simulink model "topavalon"  (Simulink 7.0)
settings: Solver=FixedStepDiscrete  StartTime=0.0  StopTime=100.0  FixedStep=1  RelTol=1e-3
InitFcn:
  | %% DSPBuilder Start
  | alt_dspbuilder_update_model(bdroot)
  | %% DSPBuilder End
undefined symbols (not defined in the file): Pin_U10, Pin_U11, Pin_U5, Pin_U6, Pin_V10, Pin_V4, Pin_V5, Pin_V6, Pin_V7, Pin_V9, Pin_W6, Pin_W7, Pin_W8, Pin_W9
libraries: allblocks_alteradspbuilder2 x33, Stratix_EP2S60_alteradspbuilder2 x3, simulink x2
settings Model: Creator=DOLSEN  LastModifiedBy=DOLSEN
settings DataIOCC: SignalLoggingName=sigsOut
settings OptimizationCC: BlockReduction=off  BooleanDataType=off
settings DebuggingCC: AlgebraicLoopMsg=none  SaveWithParameterizedLinksMsg=none  SignalResolutionControl=TryResolveAllWithWarning  SolverPrmCheckMsg=none  MultiTaskDSMMsg=warning  MultiTaskCondExecSysMsg=none
settings HardwareCC: TargetUnknown=on
settings RTWCC: IncludeERTFirstTime=on
settings GRTTargetCC: TargetFcnLib=ansi_tfl_tmw.mat  ModelReferenceCompliant=off  MatFileLogging=off

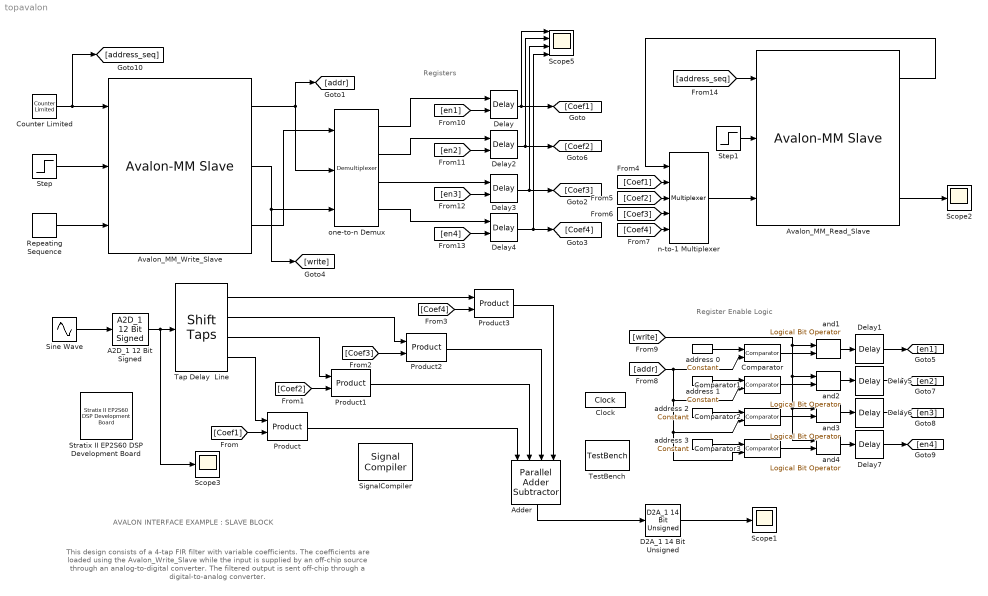
== system topavalon ==
  note: AVALON INTERFACE EXAMPLE : SLAVE BLOCK
  note: This design consists of a 4-tap FIR filter with variable coefficients.  The
      | coefficients are loaded using the Avalon_Write_Slave while the input is
      | supplied by an off-chip source through an analog-to-digital converter. The
      | filtered output is sent off-chip through a digital-to-analog converter.
  note: Register Enable Logic
  note: Registers
  A2D_1 12 Bit Signed : Stratix_EP2S60_alteradspbuilder2/A2D_1 12 Bit Signed  iofile=C:\altera\80\quartus\dsp_builder\DesignExamples\Tutorials\SOPCBuilder\SOPCBlock\My_System\tb_topavalon\topavalon_A2D%5F1+12+Bit+Signed.salt  externalType=Inferred  SpecifyClock=off  location=Pin_D1,Pin_D2 ,Pin_E3 ,Pin_E4 ,Pin_E1 ,Pin_E2 ,Pin_F3 ,Pin_F4 ,Pin_F1 ,Pin_F2 ,Pin_G3 ,Pin_G4
  Adder : allblocks_alteradspbuilder2/Parallel Adder Subtractor  Orientation=down  number_of_inputs=4  direction=++  use_pipeline=off  pipeline_display=0  phase_selection=1  use_ena=off  use_aclr=off  allowFloatingPointOverride=on  logOutputs=off  logFile=C:\altera\80\quartus\dsp_builder\DesignExamples\Tutorials\SOPCBuilder\SOPCBlock\My_System\tb_topavalon\topavalon_Adder.fixedpointlog
  Avalon_MM_Read_Slave : allblocks_alteradspbuilder2/Avalon-MM Slave  SystemSampleTime=-1  iofile=C:\altera\80\quartus\dsp_builder\DesignExamples\Tutorials\SOPCBuilder\SOPCBlock\My_System\tb_topavalon\topavalon_Avalon%5FMM%5FRead%5FSlave_address.salt,C:\altera\80\quartus\dsp_builder\DesignExamples\Tutorials\SOPCBuilder\SOPCBlock\My_System\tb_topavalon\topavalon_Avalon%5FMM%5FRead%5FSlave_read.salt,C:\altera\80\quartus\dsp_builder\DesignExamples\Tutorials\SOPCBuilder\SOPCBlock\My_System\tb_topavalon\topavalon_Avalon%5FMM%5FRead%5FSlave_readdata.capture,  SpecifyClock=off  addrWidth=2  addrAlignment=Dynamic  addrType=Read  BusType=Unsigned Integer  bwl=8  bwr=0  byteEnable=off  flowCtrl=off  pipeline=off  waitStateFormat=Fixed  readWaitStateCycles=0  writeWaitStateCycles=0  readLatencyFormat=Fixed  readLatencyCycles=0  burst=off  maxBurst=4  irq=off  receiveBeginTransfer=off  useChipSelect=off  externalType=Inferred  PORTTYPE=Output
  Avalon_MM_Write_Slave : allblocks_alteradspbuilder2/Avalon-MM Slave  SystemSampleTime=-1  iofile=C:\altera\80\quartus\dsp_builder\DesignExamples\Tutorials\SOPCBuilder\SOPCBlock\My_System\tb_topavalon\topavalon_Avalon%5FMM%5FWrite%5FSlave_address.salt,C:\altera\80\quartus\dsp_builder\DesignExamples\Tutorials\SOPCBuilder\SOPCBlock\My_System\tb_topavalon\topavalon_Avalon%5FMM%5FWrite%5FSlave_write.salt,C:\altera\80\quartus\dsp_builder\DesignExamples\Tutorials\SOPCBuilder\SOPCBlock\My_System\tb_topavalon\topavalon_Avalon%5FMM%5FWrite%5FSlave_writedata.salt,  SpecifyClock=off  addrWidth=2  addrAlignment=Dynamic  addrType=Write  BusType=Unsigned Integer  bwl=8  bwr=0  byteEnable=off  flowCtrl=off  pipeline=off  waitStateFormat=Fixed  readWaitStateCycles=0  writeWaitStateCycles=0  readLatencyFormat=Fixed  readLatencyCycles=0  burst=off  maxBurst=4  irq=off  receiveBeginTransfer=off  useChipSelect=off  externalType=Inferred  PORTTYPE=Output
  Clock : allblocks_alteradspbuilder2/Clock  ClockPeriod=100  ClockPeriodUnit=ns  SampleTime=1  SimulationStartCycle=5  PhaseOffset=0  Reset=aclr  ResetType=Active Low  Export=off
  Comparator : allblocks_alteradspbuilder2/Comparator  direction=a == b  pipeline_display=0  allowFloatingPointOverride=on  logOutputs=off  logFile=C:\altera\80\quartus\dsp_builder\DesignExamples\Tutorials\SOPCBuilder\SOPCBlock\My_System\tb_topavalon\topavalon_Comparator.fixedpointlog
  Comparator1 : allblocks_alteradspbuilder2/Comparator  direction=a == b  pipeline_display=0  allowFloatingPointOverride=on  logOutputs=off  logFile=C:\altera\80\quartus\dsp_builder\DesignExamples\Tutorials\SOPCBuilder\SOPCBlock\My_System\tb_topavalon\topavalon_Comparator1.fixedpointlog
  Comparator2 : allblocks_alteradspbuilder2/Comparator  direction=a == b  pipeline_display=0  allowFloatingPointOverride=on  logOutputs=off  logFile=C:\altera\80\quartus\dsp_builder\DesignExamples\Tutorials\SOPCBuilder\SOPCBlock\My_System\tb_topavalon\topavalon_Comparator2.fixedpointlog
  Comparator3 : allblocks_alteradspbuilder2/Comparator  direction=a == b  pipeline_display=0  allowFloatingPointOverride=on  logOutputs=off  logFile=C:\altera\80\quartus\dsp_builder\DesignExamples\Tutorials\SOPCBuilder\SOPCBlock\My_System\tb_topavalon\topavalon_Comparator3.fixedpointlog
  Counter Limited : simulink/Sources/Counter Limited  SystemSampleTime=-1  uplimit=3  tsamp=1
  D2A_1 14 Bit Unsigned : Stratix_EP2S60_alteradspbuilder2/D2A_1 14 Bit Unsigned  iofile=C:\altera\80\quartus\dsp_builder\DesignExamples\Tutorials\SOPCBuilder\SOPCBlock\My_System\tb_topavalon\topavalon_D2A%5F1+14+Bit+Unsigned.capture  externalType=Inferred  location=Pin_W7,Pin_W6,Pin_W9,Pin_W8,Pin_V5,Pin_V4,Pin_V7,Pin_V6,Pin_V10,Pin_V9,Pin_U11,Pin_U10,Pin_U6,Pin_U5
  Delay : allblocks_alteradspbuilder2/Delay  pipeline=1  pipeline_display=1  ClockPhase=1  use_ena=on  use_sclr=off  allowFloatingPointOverride=on  logOutputs=off  logFile=C:\altera\80\quartus\dsp_builder\DesignExamples\Tutorials\SOPCBuilder\SOPCBlock\My_System\tb_topavalon\topavalon_Delay.fixedpointlog  use_init=off  reset_value=1
  Delay1 : allblocks_alteradspbuilder2/Delay  pipeline=1  pipeline_display=1  ClockPhase=1  use_ena=off  use_sclr=off  allowFloatingPointOverride=on  logOutputs=off  logFile=C:\altera\80\quartus\dsp_builder\DesignExamples\Tutorials\SOPCBuilder\SOPCBlock\My_System\tb_topavalon\topavalon_Delay1.fixedpointlog  use_init=off  reset_value=1
  Delay2 : allblocks_alteradspbuilder2/Delay  pipeline=1  pipeline_display=1  ClockPhase=1  use_ena=on  use_sclr=off  allowFloatingPointOverride=on  logOutputs=off  logFile=C:\altera\80\quartus\dsp_builder\DesignExamples\Tutorials\SOPCBuilder\SOPCBlock\My_System\tb_topavalon\topavalon_Delay2.fixedpointlog  use_init=off  reset_value=1
  Delay3 : allblocks_alteradspbuilder2/Delay  pipeline=1  pipeline_display=1  ClockPhase=1  use_ena=on  use_sclr=off  allowFloatingPointOverride=on  logOutputs=off  logFile=C:\altera\80\quartus\dsp_builder\DesignExamples\Tutorials\SOPCBuilder\SOPCBlock\My_System\tb_topavalon\topavalon_Delay3.fixedpointlog  use_init=off  reset_value=1
  Delay4 : allblocks_alteradspbuilder2/Delay  pipeline=1  pipeline_display=1  ClockPhase=1  use_ena=on  use_sclr=off  allowFloatingPointOverride=on  logOutputs=off  logFile=C:\altera\80\quartus\dsp_builder\DesignExamples\Tutorials\SOPCBuilder\SOPCBlock\My_System\tb_topavalon\topavalon_Delay4.fixedpointlog  use_init=off  reset_value=1
  Delay5 : allblocks_alteradspbuilder2/Delay  pipeline=1  pipeline_display=1  ClockPhase=1  use_ena=off  use_sclr=off  allowFloatingPointOverride=on  logOutputs=off  logFile=C:\altera\80\quartus\dsp_builder\DesignExamples\Tutorials\SOPCBuilder\SOPCBlock\My_System\tb_topavalon\topavalon_Delay5.fixedpointlog  use_init=off  reset_value=1
  Delay6 : allblocks_alteradspbuilder2/Delay  pipeline=1  pipeline_display=1  ClockPhase=1  use_ena=off  use_sclr=off  allowFloatingPointOverride=on  logOutputs=off  logFile=C:\altera\80\quartus\dsp_builder\DesignExamples\Tutorials\SOPCBuilder\SOPCBlock\My_System\tb_topavalon\topavalon_Delay6.fixedpointlog  use_init=off  reset_value=1
  Delay7 : allblocks_alteradspbuilder2/Delay  pipeline=1  pipeline_display=1  ClockPhase=1  use_ena=off  use_sclr=off  allowFloatingPointOverride=on  logOutputs=off  logFile=C:\altera\80\quartus\dsp_builder\DesignExamples\Tutorials\SOPCBuilder\SOPCBlock\My_System\tb_topavalon\topavalon_Delay7.fixedpointlog  use_init=off  reset_value=1
  Product : allblocks_alteradspbuilder2/Product  BusType=Inferred  bwl=8  bwr=0  pipeline=0  pipeline_display=0  phase_selection=1  use_ena=off  use_aclr=off  UseLPM=off  UseDedicatedCircuitry=off  allowFloatingPointOverride=on  logOutputs=off  logFile=C:\altera\80\quartus\dsp_builder\DesignExamples\Tutorials\SOPCBuilder\SOPCBlock\My_System\tb_topavalon\topavalon_Product.fixedpointlog
  Product1 : allblocks_alteradspbuilder2/Product  BusType=Inferred  bwl=8  bwr=0  pipeline=0  pipeline_display=0  phase_selection=1  use_ena=off  use_aclr=off  UseLPM=off  UseDedicatedCircuitry=off  allowFloatingPointOverride=on  logOutputs=off  logFile=C:\altera\80\quartus\dsp_builder\DesignExamples\Tutorials\SOPCBuilder\SOPCBlock\My_System\tb_topavalon\topavalon_Product1.fixedpointlog
  Product2 : allblocks_alteradspbuilder2/Product  BusType=Inferred  bwl=8  bwr=0  pipeline=0  pipeline_display=0  phase_selection=1  use_ena=off  use_aclr=off  UseLPM=off  UseDedicatedCircuitry=off  allowFloatingPointOverride=on  logOutputs=off  logFile=C:\altera\80\quartus\dsp_builder\DesignExamples\Tutorials\SOPCBuilder\SOPCBlock\My_System\tb_topavalon\topavalon_Product2.fixedpointlog
  Product3 : allblocks_alteradspbuilder2/Product  BusType=Inferred  bwl=8  bwr=0  pipeline=0  pipeline_display=0  phase_selection=1  use_ena=off  use_aclr=off  UseLPM=off  UseDedicatedCircuitry=off  allowFloatingPointOverride=on  logOutputs=off  logFile=C:\altera\80\quartus\dsp_builder\DesignExamples\Tutorials\SOPCBuilder\SOPCBlock\My_System\tb_topavalon\topavalon_Product3.fixedpointlog
  Repeating Sequence : simulink/Sources/Repeating Sequence  SystemSampleTime=-1  rep_seq_t=[0 1 2 3 4]  rep_seq_y=[1 0 0 0 0]
  Scope1 : Scope
      settings: SampleInput=on
  Scope2 : Scope
      settings: SampleInput=on
  Scope3 : Scope
      settings: SaveName=ScopeData2  SampleInput=on
  Scope5 : Scope  NumInputPorts=4
      settings: TimeRange=100  YMin=0~0~0~-1  YMax=1~1~1~1  SaveName=ScopeData3  SampleInput=on
  SignalCompiler : allblocks_alteradspbuilder2/Signal Compiler  DeviceFamily=Stratix II  DeviceName=EP2S60F1020C4ES  EnableSignalTap=off  SignalTapDepth=128  UseBoardBlock=off  StpUseDefaultClock=on  StpClock=Clock  ExportDir=C:\Documents and Settings\dolsen\My Documents
  Sine Wave : Sin  Amplitude=2^11-1  SampleTime=1
  Step : Step  Time=4  Before=1  After=0  SampleTime=1
  Step1 : Step  Time=10  Before=1  After=0  SampleTime=1
  Stratix II EP2S60 DSP Development Board : Stratix_EP2S60_alteradspbuilder2/Stratix II EP2S60 DSP Development Board  ClockPinIn=Pin_AM17  GlobalResetPin=Pin_AG19  device=EP2S60F1020C4
  Tap Delay  Line : allblocks_alteradspbuilder2/Shift Taps  number_of_taps=4  tap_distance=1  use_shiftout=off  use_ena=off  use_sclr=off  use_dedicated_circuitry=on  ram_type=AUTO  allowFloatingPointOverride=on  logOutputs=off  logFile=C:\altera\80\quartus\dsp_builder\DesignExamples\Tutorials\SOPCBuilder\SOPCBlock\My_System\tb_topavalon\topavalon_Tap+Delay+%0ALine%3A%3At.fixedpointlog,C:\altera\80\quartus\dsp_builder\DesignExamples\Tutorials\SOPCBuilder\SOPCBlock\My_System\tb_topavalon\topavalon_Tap+Delay+%0ALine%3A%3At.fixedpointlog,C:\altera\80\quartus\dsp_builder\DesignExamples\Tutorials\SOPCBuilder\SOPCBlock\My_System\tb_topavalon\topavalon_Tap+Delay+%0ALine%3A%3At.fixedpointlog,C:\altera\80\quartus\dsp_builder\DesignExamples\Tutorials\SOPCBuilder\SOPCBlock\My_System\tb_topavalon\topavalon_Tap+Delay+%0ALine%3A%3At.fixedpointlog,
  TestBench : allblocks_alteradspbuilder2/TestBench  enable=on  advancedMode=off  modelSimGui=off  maxDisplayErrors=10  mismatchErrorLevel=Error  simdatafile=C:\altera\80\quartus\dsp_builder\DesignExamples\Tutorials\SOPCBuilder\SOPCBlock\My_System\tb_topavalon\topavalon.simdata.tcl
  address 0 : allblocks_alteradspbuilder2/Constant  mask_cst=0  BusType=Unsigned Integer  bwl=2  bwr=0  roundMode=Truncate  satMode=Wrap  SpecifyClock=off  allowFloatingPointOverride=on  logOutputs=off  logFile=C:\altera\80\quartus\dsp_builder\DesignExamples\Tutorials\SOPCBuilder\SOPCBlock\My_System\tb_topavalon\topavalon_address+0.fixedpointlog
  address 1 : allblocks_alteradspbuilder2/Constant  mask_cst=1  BusType=Unsigned Integer  bwl=2  bwr=0  roundMode=Truncate  satMode=Wrap  SpecifyClock=off  allowFloatingPointOverride=on  logOutputs=off  logFile=C:\altera\80\quartus\dsp_builder\DesignExamples\Tutorials\SOPCBuilder\SOPCBlock\My_System\tb_topavalon\topavalon_address+1.fixedpointlog
  address 2 : allblocks_alteradspbuilder2/Constant  mask_cst=2  BusType=Unsigned Integer  bwl=2  bwr=0  roundMode=Truncate  satMode=Wrap  SpecifyClock=off  allowFloatingPointOverride=on  logOutputs=off  logFile=C:\altera\80\quartus\dsp_builder\DesignExamples\Tutorials\SOPCBuilder\SOPCBlock\My_System\tb_topavalon\topavalon_address+2.fixedpointlog
  address 3 : allblocks_alteradspbuilder2/Constant  mask_cst=3  BusType=Unsigned Integer  bwl=2  bwr=0  roundMode=Truncate  satMode=Wrap  SpecifyClock=off  allowFloatingPointOverride=on  logOutputs=off  logFile=C:\altera\80\quartus\dsp_builder\DesignExamples\Tutorials\SOPCBuilder\SOPCBlock\My_System\tb_topavalon\topavalon_address+3.fixedpointlog
  and{1..4} (4 alike) : allblocks_alteradspbuilder2/Logical Bit Operator  LogicalOperator=AND  user_inputs=2  pipeline_display=0
  n-to-1 Multiplexer : allblocks_alteradspbuilder2/Multiplexer  numInputs=4  pipeline=0  oneHot=off  pipeline_display=0  use_ena=off  use_aclr=off  allowFloatingPointOverride=on  logOutputs=off  logFile=C:\altera\80\quartus\dsp_builder\DesignExamples\Tutorials\SOPCBuilder\SOPCBlock\My_System\tb_topavalon\topavalon_n-to-1+Multiplexer.fixedpointlog
  one-to-n Demux : allblocks_alteradspbuilder2/Demultiplexer  numOutputs=4  pipeline_display=1  use_ena=on  use_sclr=off  allowFloatingPointOverride=on  logOutputs=off  logFile=C:\altera\80\quartus\dsp_builder\DesignExamples\Tutorials\SOPCBuilder\SOPCBlock\My_System_\tb_topavalon\topavalon_one-to-n+Demux%3A%3Aq.fixedpointlog,C:\altera\80\quartus\dsp_builder\DesignExamples\Tutorials\SOPCBuilder\SOPCBlock\My_System_\tb_topavalon\topavalon_one-to-n+Demux%3A%3Aq.fixedpointlog,C:\altera\80\quartus\dsp_builder\DesignExamples\Tutorials\SOPCBuilder\SOPCBlock\My_System_\tb_topavalon\topavalon_one-to-n+Demux%3A%3Aq.fixedpointlog,C:\altera\80\quartus\dsp_builder\DesignExamples\Tutorials\SOPCBuilder\SOPCBlock\My_System_\tb_topavalon\topavalon_one-to-n+Demux%3A%3Aq.fixedpointlog,
  wires:
  Tap Delay  Line/4 -> Product/1
  Tap Delay  Line/3 -> Product1/1
  Tap Delay  Line/2 -> Product2/1
  Tap Delay  Line/1 -> Product3/1
  Product/1 -> Adder/1
  A2D_1 12 Bit Signed/1 -> Tap Delay  Line/1, Scope3/1
  Product1/1 -> Adder/2
  Product2/1 -> Adder/3
  Product3/1 -> Adder/4
  Adder/1 -> D2A_1 14 Bit Unsigned/1
  [Coef1] -> Product/2
  [Coef2] -> Product1/2
  [Coef3] -> Product2/2
  [Coef4] -> Product3/2
  one-to-n Demux/1 -> Delay/1
  one-to-n Demux/2 -> Delay2/1
  one-to-n Demux/3 -> Delay3/1
  one-to-n Demux/4 -> Delay4/1
  Avalon_MM_Write_Slave/1 -> one-to-n Demux/2, [addr]
  Avalon_MM_Write_Slave/2 -> one-to-n Demux/3, [write]
  Avalon_MM_Write_Slave/3 -> one-to-n Demux/1
  n-to-1 Multiplexer/1 -> Avalon_MM_Read_Slave/3
  Sine Wave/1 -> A2D_1 12 Bit Signed/1
  address 0/1 -> Comparator/1
  address 1/1 -> Comparator1/1
  address 2/1 -> Comparator2/1
  address 3/1 -> Comparator3/1
  Comparator/1 -> and1/2
  Comparator1/1 -> and2/2
  Comparator2/1 -> and3/2
  Comparator3/1 -> and4/2
  [write] -> and3/1, and4/1, and2/1, and1/1
  and1/1 -> Delay1/1
  and2/1 -> Delay5/1
  and3/1 -> Delay6/1
  and4/1 -> Delay7/1
  [en1] -> Delay/2
  [en2] -> Delay2/2
  [en3] -> Delay3/2
  [en4] -> Delay4/2
  Delay1/1 -> [en1]
  Delay5/1 -> [en2]
  Delay6/1 -> [en3]
  Delay7/1 -> [en4]
  [addr] -> Comparator/2, Comparator1/2, Comparator2/2, Comparator3/2
  D2A_1 14 Bit Unsigned/1 -> Scope1/1
  Avalon_MM_Read_Slave/1 -> n-to-1 Multiplexer/1
  [Coef1] -> n-to-1 Multiplexer/2
  [Coef2] -> n-to-1 Multiplexer/3
  [Coef3] -> n-to-1 Multiplexer/4
  [Coef4] -> n-to-1 Multiplexer/5
  Counter Limited/1 -> [address_seq], Avalon_MM_Write_Slave/1
  Step/1 -> Avalon_MM_Write_Slave/2
  Repeating Sequence/1 -> Avalon_MM_Write_Slave/3
  Avalon_MM_Read_Slave/3 -> Scope2/1
  [address_seq] -> Avalon_MM_Read_Slave/1
  Step1/1 -> Avalon_MM_Read_Slave/2
  Delay/1 -> Scope5/1, [Coef1]
  Delay2/1 -> Scope5/2, [Coef2]
  Delay3/1 -> Scope5/3, [Coef3]
  Delay4/1 -> Scope5/4, [Coef4]
